simulink model "tractionControlSystem1"  (R2018b)
settings: Solver=ode45  StartTime=0.0  StopTime=10.0  MinStep=0.001  RelTol=1e-6  EnableMultiTasking=on
values from neighbouring files (symbols this model uses):
  be = 0.008    [parameter.m]
  driverDesired = 180    [parameter.m]
  Je = 0.28    [parameter.m]
  m = 1631    [parameter.m]
  R = 0.12055    [parameter.m]
  r_e = 0.35    [parameter.m]
  sigma_max = % Fill with answer from 1.1    [parameter.m]
  tau_f = 0.004    [parameter.m]
undefined symbols (not defined in the file or in its folder): arrFl, arrSigma
libraries: simulink x1
settings Model: Creator=YW Liao  LastModifiedBy=trey
settings DataIOCC: LimitDataPoints=on  SaveFormat=Array
settings OptimizationCC: LifeSpan=inf
settings DebuggingCC: UnderspecifiedInitializationDetection=Classic  MergeDetectMultiDrivingBlocksExec=none  SolverPrmCheckMsg=warning  StateNameClashWarn=warning  SFUnexpectedBacktrackingDiag=warning  SFNoUnconditionalDefaultTransitionDiag=warning  SFExecutionAtInitializationDiag=none
settings HardwareCC: ProdBitPerPointer=32  ProdBitPerSizeT=32  ProdBitPerPtrDiffT=32  ProdLargestAtomicFloat=None  ProdIntDivRoundTo=Undefined  ProdEndianess=Unspecified  ProdWordSize=32  ProdHWDeviceType=32-bit Generic
settings ModelReferenceCC: PropagateSignalLabelsOutOfModel=off
settings SFSimCC: SimUseLocalCustomCode=off
settings RTWCC: RTWUseLocalCustomCode=off
settings CodeAppCC: StateflowObjectComments=on
settings GRTTargetCC: TargetLangStandard=C89/C90 (ANSI)  GeneratePreprocessorConditionals=Disable all
settings ConfigComp: CovMetricSettings=dw  CovHtmlReporting=on  CovSaveCumulativeToWorkspaceVar=on  CovSaveSingleToWorkspaceVar=on  CovExternalEMLEnable=off
settings SimscapeCC: SimscapeNormalizeSystem=off
settings ConfigurationSet: Description=SimMechanics 2G

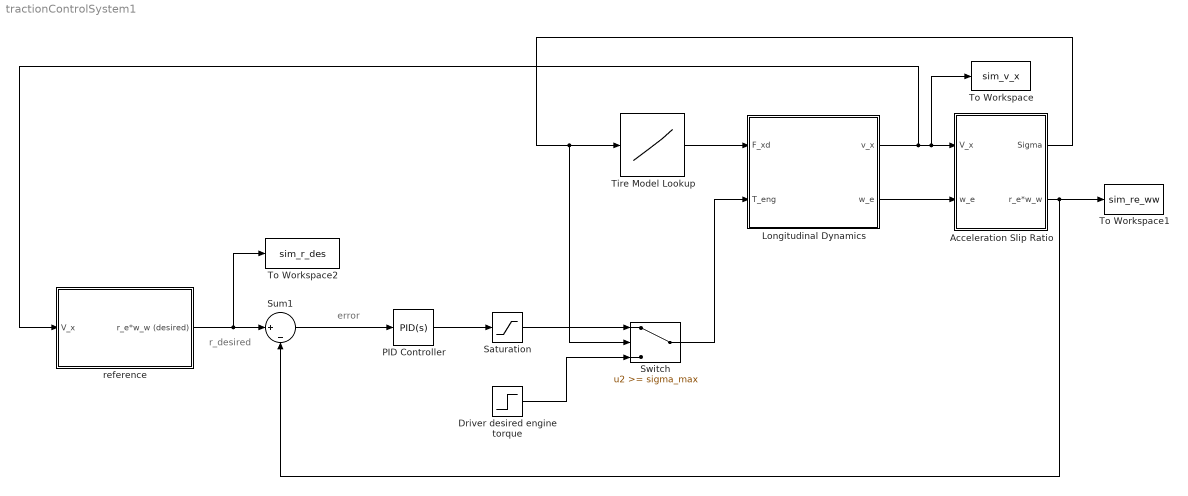
== system tractionControlSystem1 ==
  note: error
  note: r_desired
  Acceleration Slip Ratio : Subsystem
  Driver desired engine torque : Step  Time=0  After=driverDesired  SampleTime=0
  Longitudinal Dynamics : Subsystem
  "PID Controller " : simulink/Continuous/PID Controller  Controller=PID  Form=Parallel  TimeDomain=Continuous-time  SampleTime=-1  IntegratorMethod=Forward Euler  FilterMethod=Forward Euler  ControllerParametersSource=internal  P=300  I=500  D=0  UseFilter=on  N=100  TunerSelectOption=Transfer Function Based (PID Tuner App)  InitialConditionSource=internal  InitialConditionForIntegrator=0  InitialConditionForFilter=0  DifferentiatorICPrevScaledInput=0  ExternalReset=none  TrackingMode=off  Kt=1  LimitOutput=off  UpperSaturationLimit=inf  LowerSaturationLimit=-inf  LinearizeAsGain=on  AntiWindupMode=none  Kb=1  POutMin=[]  POutMax=[]  IOutMin=[]  IOutMax=[]  DOutMin=[]  DOutMax=[]  NOutMin=[]  NOutMax=[]  SumOutMin=[]  SumOutMax=[]  SaturationOutMin=[]  SaturationOutMax=[]  PParamMin=[]  PParamMax=[]  IParamMin=[]  IParamMax=[]  DParamMin=[]  DParamMax=[]  NParamMin=[]  NParamMax=[]  KbParamMin=[]  KbParamMax=[]  KtParamMin=[]  KtParamMax=[]  KbOutMin=[]  KbOutMax=[]  KtOutMin=[]  KtOutMax=[]  IntegratorOutMin=[]  IntegratorOutMax=[]  FilterOutMin=[]  FilterOutMax=[]  SumI1OutMin=[]  SumI1OutMax=[]  SumI2OutMin=[]  SumI2OutMax=[]  SumI3OutMin=[]  SumI3OutMax=[]  SumI4OutMin=[]  SumI4OutMax=[]  SumDOutMin=[]  SumDOutMax=[]  DifferentiatorOutMin=[]  DifferentiatorOutMax=[]  FilterDiffOutCoefMin=[]  FilterDiffOutCoefMax=[]  ReciprocalOutMin=[]  ReciprocalOutMax=[]  SumDenOutMin=[]  SumDenOutMax=[]  SumNumOutMin=[]  SumNumOutMax=[]  DivideOutMin=[]  DivideOutMax=[]  IntegratorContinuousStateAttributes=''  IntegratorStateMustResolveToSignalObject=off  IntegratorRTWStateStorageClass=Auto  FilterContinuousStateAttributes=''  FilterStateMustResolveToSignalObject=off  FilterRTWStateStorageClass=Auto  ParallelPVariant=InternalParameters  IdealPVariant=Disabled  IVariant=InternalParameters  DVariant=InternalParameters  IntegratorVariant=Continuous  SatVariant=Disabled  AWVariant=Passthrough  PCopyVariant=Disabled  TRVariant=Disabled  FdbkBlocksVariant=Forward  IdealPFdbkVariant=Disabled  SatFdbkVariant=Disabled  DerivativeFilterVariant=ContFilter  NVariant=InternalParameters  NCopyVariant=Disabled  FilterICVariant=InternalICsFilter  IntegratorICVariant=InternalICs  ExternalResetVariant=Disabled  TRSumVariant=Passthrough  SumFdbkVariant=Disabled  SumVariant=Sum_PID
  Saturation : Saturate  UpperLimit=180  LowerLimit=-30
  Sum1 : Sum  Inputs=||+|-
  Switch : Switch  Threshold=sigma_max  ZeroCross=off
  Tire Model Lookup : Lookup_n-D  NumberOfTableDimensions=1  LookupTableObject=tireForceModel  BreakpointsForDimension1=arrSigma  Table=arrFl  InternalRulePriority=Speed  RndMeth=Simplest  InputSameDT=on
  To Workspace : ToWorkspace  VariableName=sim_v_x  SaveFormat=Timeseries  SampleTime=-1
  To Workspace1 : ToWorkspace  VariableName=sim_re_ww  SaveFormat=Timeseries  SampleTime=-1
  To Workspace2 : ToWorkspace  VariableName=sim_r_des  SaveFormat=Timeseries  SampleTime=-1
  reference : Subsystem
  wires:
  Sum1/1 -> "PID Controller "/1
  Longitudinal Dynamics/1(v_x) -> To Workspace/1, Acceleration Slip Ratio/1(V_x), reference/1(V_x)
  "PID Controller "/1 -> Saturation/1
  Longitudinal Dynamics/2(w_e) -> Acceleration Slip Ratio/2(w_e)
  Driver desired engine torque/1 -> Switch/3
  Saturation/1 -> Switch/1
  Switch/1 -> Longitudinal Dynamics/2(T_eng)
  Acceleration Slip Ratio/2(r_e*w_w) -> Sum1/2, To Workspace1/1
  reference/1(r_e*w_w (desired)) -> To Workspace2/1, Sum1/1
  Acceleration Slip Ratio/1(Sigma) -> Tire Model Lookup/1, Switch/2
  Tire Model Lookup/1 -> Longitudinal Dynamics/1(F_xd)

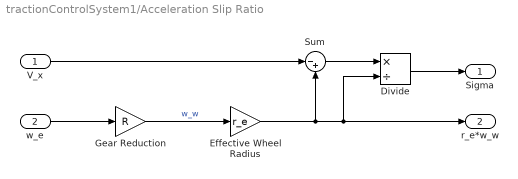
== system tractionControlSystem1/Acceleration Slip Ratio ==
  V_x : Inport
  w_e : Inport  Port=2
  Divide : Product  Inputs=*/
  Effective Wheel Radius : Gain  Gain=r_e
  Gear Reduction : Gain  Gain=R
  Sum : Sum  Inputs=|-+
  Sigma : Outport
  r_e*w_w : Outport  Port=2
  wires:
  w_e/1 -> Gear Reduction/1
  Gear Reduction/1 -> Effective Wheel Radius/1  "w_w"
  Effective Wheel Radius/1 -> Sum/2, Divide/2, r_e*w_w/1
  V_x/1 -> Sum/1
  Sum/1 -> Divide/1
  Divide/1 -> Sigma/1

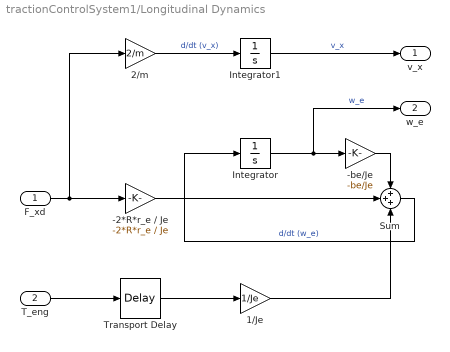
== system tractionControlSystem1/Longitudinal Dynamics ==
  F_xd : Inport
  T_eng : Inport  Port=2
  -2*R*r_e / Je : Gain  Gain=-2*R*r_e / Je
  -be/Je : Gain  Gain=-be/Je
  1/Je : Gain  Gain=1/Je
  2/m : Gain  Gain=2/m
  Integrator : Integrator  InitialCondition=0.001 / (r_e*R)
  Integrator1 : Integrator  InitialCondition=0.001
  Sum : Sum  Inputs=+++
  Transport Delay : TransportDelay  DelayTime=tau_f
  v_x : Outport
  w_e : Outport  Port=2
  wires:
  Integrator/1 -> w_e/1, -be/Je/1  "w_e"
  T_eng/1 -> Transport Delay/1
  Transport Delay/1 -> 1/Je/1
  F_xd/1 -> 2/m/1, -2*R*r_e / Je/1
  -2*R*r_e / Je/1 -> Sum/2
  1/Je/1 -> Sum/3
  -be/Je/1 -> Sum/1
  Sum/1 -> Integrator/1  "d/dt (w_e)"
  2/m/1 -> Integrator1/1  "d/dt (v_x)"
  Integrator1/1 -> v_x/1  "v_x"

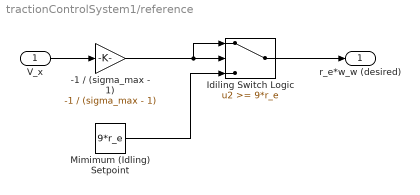
== system tractionControlSystem1/reference ==
  V_x : Inport
  -1 / (sigma_max - 1) : Gain  Gain=-1 / (sigma_max - 1)
  Idiling Switch Logic : Switch  Threshold=9*r_e
  Mimimum (Idling) Setpoint : Constant  Value=9*r_e
  r_e*w_w (desired) : Outport
  wires:
  V_x/1 -> -1 / (sigma_max - 1)/1
  -1 / (sigma_max - 1)/1 -> Idiling Switch Logic/1, Idiling Switch Logic/2
  Mimimum (Idling) Setpoint/1 -> Idiling Switch Logic/3
  Idiling Switch Logic/1 -> r_e*w_w (desired)/1
